simulink model "single_integrator_formation_control"  (R2021b)
settings: Solver=ode4  StartTime=0.0  StopTime=10  FixedStep=0.1  RelTol=1e-3
values from neighbouring files (symbols this model uses):
  A = A - diag(diag(A))    [formation_params.m]
  central_bot_idx = 5    [formation_params.m]
  init_positions = init_positions + init_position_perturbation    [formation_params.m]
  num_bots = 5    [formation_params.m]
  static_formation = [0.0, 0.0, 0.0 ... (first row only)    [formation_params.m]
libraries: robotcorelib x1
settings Model: Creator=root  LastModifiedBy=NEELAKSH SINGH

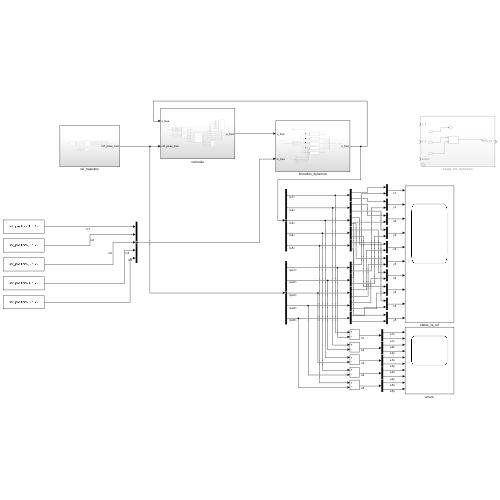
[thumbnail: Simulink's stored preview of the top-level diagram]
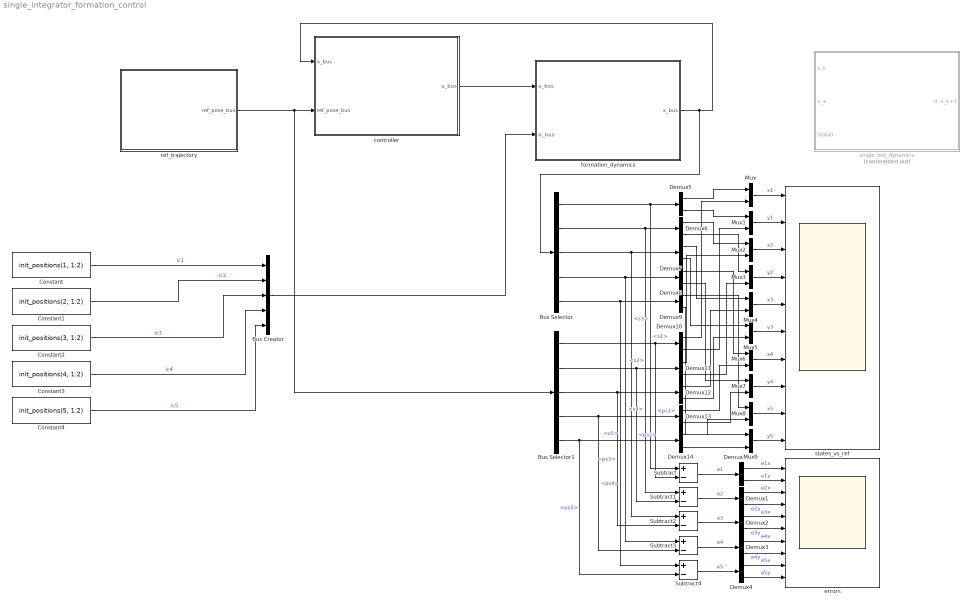
== system single_integrator_formation_control ==
  Bus Creator : BusCreator  Inputs=5
  Bus Selector : BusSelector  OutputSignals=s1,s2,s3,s4,s5
  Bus Selector1 : BusSelector  OutputSignals=ps1,ps2,ps3,ps4,ps5
  Constant : Constant  Value=init_positions(1, 1:2)
  Constant1 : Constant  Value=init_positions(2, 1:2)
  Constant2 : Constant  Value=init_positions(3, 1:2)
  Constant3 : Constant  Value=init_positions(4, 1:2)
  Constant4 : Constant  Value=init_positions(5, 1:2)
  Demux{,1..14} (15 alike) : Demux  Outputs=2
  Mux{,1..9} (10 alike) : Mux  Inputs=2
  Subtract{,1..4} (5 alike) : Sum  Inputs=+-
  controller : Subsystem
  errors : Scope  NumInputPorts=10
  formation_dynamics : Subsystem
  ref_trajectory : Subsystem
  single_bot_dynamics : Subsystem  Commented=on
  states_vs_ref : Scope  NumInputPorts=10
  wires:
  controller/1(u_bus) -> formation_dynamics/1(u_bus)
  formation_dynamics/1(x_bus) -> Bus Selector/1, controller/1(x_bus)
  Constant/1 -> Bus Creator/1  "ic1"
  Constant1/1 -> Bus Creator/2  "ic2"
  Constant2/1 -> Bus Creator/3  "ic3"
  Constant3/1 -> Bus Creator/4  "ic4"
  Constant4/1 -> Bus Creator/5  "ic5"
  Bus Creator/1 -> formation_dynamics/2(ic_bus)
  ref_trajectory/1(ref_pose_bus) -> Bus Selector1/1, controller/2(ref_pose_bus)
  Bus Selector/1 -> Demux5/1, Subtract/1  "<s1>"
  Bus Selector/2 -> Subtract1/1, Demux6/1  "<s2>"
  Bus Selector/3 -> Demux7/1, Subtract2/1  "<s3>"
  Bus Selector/4 -> Demux8/1, Subtract3/1  "<s4>"
  Bus Selector/5 -> Subtract4/1, Demux9/1  "<s5>"
  Bus Selector1/1 -> Demux10/1, Subtract/2  "<ps1>"
  Bus Selector1/2 -> Demux11/1, Subtract1/2  "<ps2>"
  Bus Selector1/3 -> Demux12/1, Subtract2/2  "<ps3>"
  Bus Selector1/4 -> Demux13/1, Subtract3/2  "<ps4>"
  Bus Selector1/5 -> Demux14/1, Subtract4/2  "<ps5>"
  Subtract4/1 -> Demux4/1  "e5"
  Subtract3/1 -> Demux3/1  "e4"
  Subtract2/1 -> Demux2/1  "e3"
  Subtract1/1 -> Demux1/1  "e2"
  Subtract/1 -> Demux/1  "e1"
  Demux/1 -> errors/1  "e1x"
  Demux4/2 -> errors/10  "e5y"
  Demux4/1 -> errors/9  "e5x"
  Demux3/1 -> errors/7  "e4x"
  Demux3/2 -> errors/8  "e4y"
  Demux2/2 -> errors/6  "e3y"
  Demux2/1 -> errors/5  "e3x"
  Demux1/2 -> errors/4  "e2y"
  Demux1/1 -> errors/3  "e2x"
  Demux/2 -> errors/2  "e1y"
  Demux5/1 -> Mux/1
  Demux10/1 -> Mux/2
  Demux5/2 -> Mux1/1
  Demux10/2 -> Mux1/2
  Demux6/1 -> Mux2/1
  Demux11/1 -> Mux2/2
  Demux6/2 -> Mux3/1
  Demux11/2 -> Mux3/2
  Demux7/1 -> Mux4/1
  Demux12/1 -> Mux4/2
  Demux7/2 -> Mux5/1
  Demux12/2 -> Mux5/2
  Demux8/1 -> Mux6/1
  Demux13/1 -> Mux6/2
  Demux8/2 -> Mux7/1
  Demux13/2 -> Mux7/2
  Demux9/1 -> Mux8/1
  Demux14/1 -> Mux8/2
  Demux9/2 -> Mux9/1
  Demux14/2 -> Mux9/2
  Mux/1 -> states_vs_ref/1  "x1"
  Mux1/1 -> states_vs_ref/2  "y1"
  Mux2/1 -> states_vs_ref/3  "x2"
  Mux3/1 -> states_vs_ref/4  "y2"
  Mux4/1 -> states_vs_ref/5  "x3"
  Mux5/1 -> states_vs_ref/6  "y3"
  Mux6/1 -> states_vs_ref/7  "x4"
  Mux7/1 -> states_vs_ref/8  "y4"
  Mux8/1 -> states_vs_ref/9  "x5"
  Mux9/1 -> states_vs_ref/10  "y5"

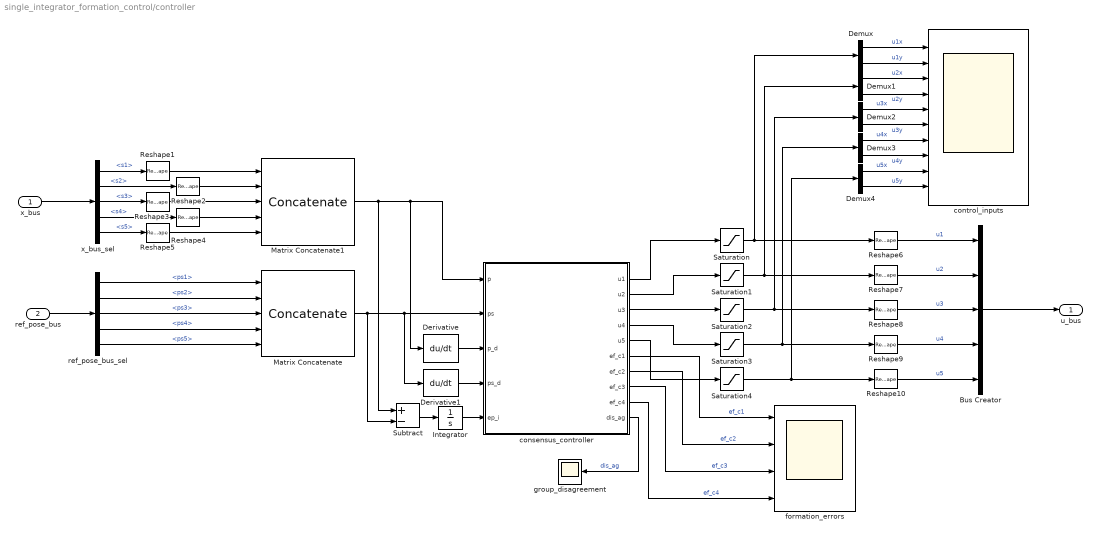
== system single_integrator_formation_control/controller ==
  x_bus : Inport
  ref_pose_bus : Inport  Port=2
  Bus Creator : BusCreator  Inputs=5
  Demux{,1..4} (5 alike) : Demux  Outputs=2
  Derivative : Derivative
  Derivative1 : Derivative
  Integrator : Integrator
  Matrix Concatenate : Concatenate  NumInputs=5  Mode=Multidimensional array  ConcatenateDimension=2
  Matrix Concatenate1 : Concatenate  NumInputs=5  Mode=Multidimensional array  ConcatenateDimension=2
  Reshape{1..10} (10 alike) : Reshape  OutputDimensionality=Column vector (2-D)
  Saturation{,1..4} (5 alike) : Saturate  UpperLimit=1  LowerLimit=-1
  Subtract : Sum  Inputs=+-
  consensus_controller : MATLAB Function  TreatAsAtomicUnit=on
  control_inputs : Scope  NumInputPorts=10
  formation_errors : Scope  NumInputPorts=4
  group_disagreement : Scope
  ref_pose_bus_sel : BusSelector  OutputSignals=ps1,ps2,ps3,ps4,ps5
  x_bus_sel : BusSelector  OutputSignals=s1,s2,s3,s4,s5
  u_bus : Outport
  wires:
  Bus Creator/1 -> u_bus/1
  consensus_controller/1(u1) -> Saturation/1
  consensus_controller/2(u2) -> Saturation1/1
  consensus_controller/3(u3) -> Saturation2/1
  consensus_controller/4(u4) -> Saturation3/1
  consensus_controller/5(u5) -> Saturation4/1
  x_bus_sel/1 -> Reshape1/1  "<s1>"
  x_bus_sel/2 -> Reshape2/1  "<s2>"
  x_bus_sel/3 -> Reshape3/1  "<s3>"
  x_bus_sel/4 -> Reshape4/1  "<s4>"
  x_bus_sel/5 -> Reshape5/1  "<s5>"
  ref_pose_bus/1 -> ref_pose_bus_sel/1
  Reshape6/1 -> Bus Creator/1  "u1"
  Reshape7/1 -> Bus Creator/2  "u2"
  Reshape8/1 -> Bus Creator/3  "u3"
  Reshape9/1 -> Bus Creator/4  "u4"
  Reshape10/1 -> Bus Creator/5  "u5"
  consensus_controller/9(ef_c4) -> formation_errors/4  "ef_c4"
  consensus_controller/6(ef_c1) -> formation_errors/1  "ef_c1"
  consensus_controller/7(ef_c2) -> formation_errors/2  "ef_c2"
  consensus_controller/8(ef_c3) -> formation_errors/3  "ef_c3"
  Demux4/2 -> control_inputs/10  "u5y"
  Demux/1 -> control_inputs/1  "u1x"
  Demux/2 -> control_inputs/2  "u1y"
  Demux1/1 -> control_inputs/3  "u2x"
  Demux1/2 -> control_inputs/4  "u2y"
  Demux2/1 -> control_inputs/5  "u3x"
  Demux2/2 -> control_inputs/6  "u3y"
  Demux3/1 -> control_inputs/7  "u4x"
  Demux3/2 -> control_inputs/8  "u4y"
  Demux4/1 -> control_inputs/9  "u5x"
  Saturation/1 -> Demux/1, Reshape6/1
  Saturation1/1 -> Demux1/1, Reshape7/1
  Saturation2/1 -> Demux2/1, Reshape8/1
  Saturation3/1 -> Demux3/1, Reshape9/1
  Saturation4/1 -> Demux4/1, Reshape10/1
  ref_pose_bus_sel/1 -> Matrix Concatenate/1  "<ps1>"
  ref_pose_bus_sel/2 -> Matrix Concatenate/2  "<ps2>"
  ref_pose_bus_sel/3 -> Matrix Concatenate/3  "<ps3>"
  ref_pose_bus_sel/4 -> Matrix Concatenate/4  "<ps4>"
  ref_pose_bus_sel/5 -> Matrix Concatenate/5  "<ps5>"
  Matrix Concatenate/1 -> Subtract/2, Derivative1/1, consensus_controller/2(ps)
  Reshape2/1 -> Matrix Concatenate1/2
  Reshape4/1 -> Matrix Concatenate1/4
  Reshape1/1 -> Matrix Concatenate1/1
  Reshape3/1 -> Matrix Concatenate1/3
  Reshape5/1 -> Matrix Concatenate1/5
  Matrix Concatenate1/1 -> consensus_controller/1(p), Derivative/1, Subtract/1
  x_bus/1 -> x_bus_sel/1
  Derivative/1 -> consensus_controller/3(p_d)
  Derivative1/1 -> consensus_controller/4(ps_d)
  Subtract/1 -> Integrator/1
  Integrator/1 -> consensus_controller/5(ep_i)
  consensus_controller/10(dis_ag) -> group_disagreement/1  "dis_ag"

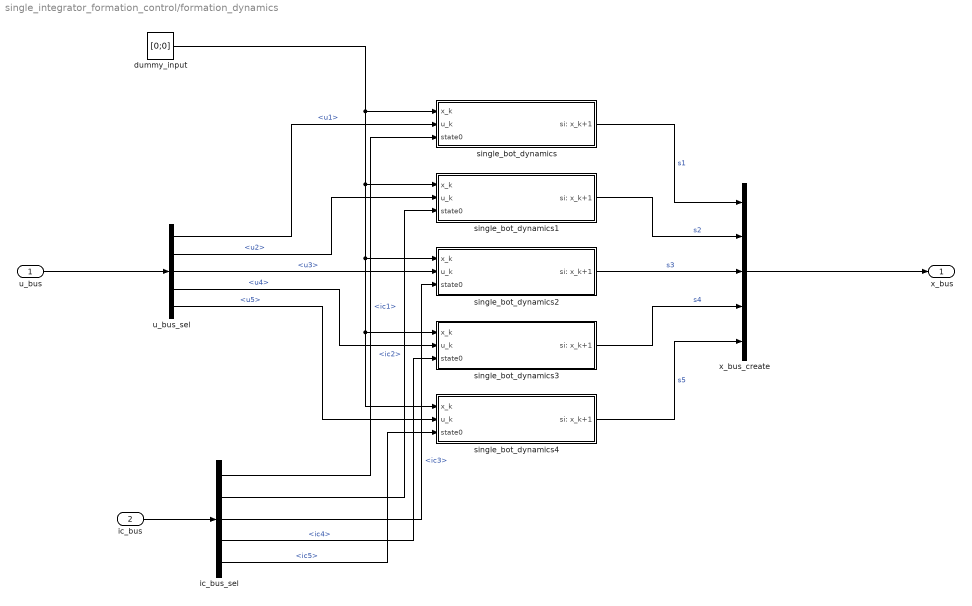
== system single_integrator_formation_control/formation_dynamics ==
  u_bus : Inport
  ic_bus : Inport  Port=2
  dummy_input : Constant  Value=[0;0]
  ic_bus_sel : BusSelector  OutputSignals=ic1,ic2,ic3,ic4,ic5
  single_bot_dynamics : Subsystem
  single_bot_dynamics1 : Subsystem
  single_bot_dynamics2 : Subsystem
  single_bot_dynamics3 : Subsystem
  single_bot_dynamics4 : Subsystem
  u_bus_sel : BusSelector  OutputSignals=u1,u2,u3,u4,u5
  x_bus_create : BusCreator  Inputs=5
  x_bus : Outport
  wires:
  u_bus_sel/1 -> single_bot_dynamics/2(u_k)  "<u1>"
  u_bus_sel/2 -> single_bot_dynamics1/2(u_k)  "<u2>"
  u_bus_sel/3 -> single_bot_dynamics2/2(u_k)  "<u3>"
  u_bus_sel/4 -> single_bot_dynamics3/2(u_k)  "<u4>"
  u_bus_sel/5 -> single_bot_dynamics4/2(u_k)  "<u5>"
  single_bot_dynamics1/1(si: x_k+1) -> x_bus_create/2  "s2"
  single_bot_dynamics2/1(si: x_k+1) -> x_bus_create/3  "s3"
  single_bot_dynamics3/1(si: x_k+1) -> x_bus_create/4  "s4"
  single_bot_dynamics4/1(si: x_k+1) -> x_bus_create/5  "s5"
  ic_bus/1 -> ic_bus_sel/1
  ic_bus_sel/1 -> single_bot_dynamics/3(state0)  "<ic1>"
  ic_bus_sel/2 -> single_bot_dynamics1/3(state0)  "<ic2>"
  ic_bus_sel/3 -> single_bot_dynamics2/3(state0)  "<ic3>"
  ic_bus_sel/4 -> single_bot_dynamics3/3(state0)  "<ic4>"
  ic_bus_sel/5 -> single_bot_dynamics4/3(state0)  "<ic5>"
  u_bus/1 -> u_bus_sel/1
  x_bus_create/1 -> x_bus/1
  single_bot_dynamics/1(si: x_k+1) -> x_bus_create/1  "s1"
  dummy_input/1 -> single_bot_dynamics4/1(x_k), single_bot_dynamics3/1(x_k), single_bot_dynamics2/1(x_k), single_bot_dynamics1/1(x_k), single_bot_dynamics/1(x_k)

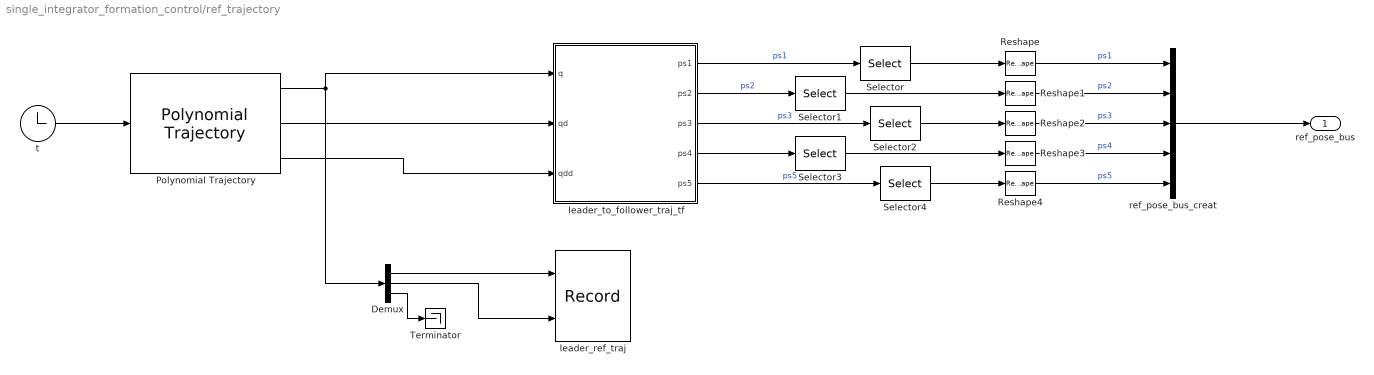
== system single_integrator_formation_control/ref_trajectory ==
  Demux : Demux  Outputs=3
  Polynomial Trajectory : robotcorelib/Polynomial Trajectory  WaypointSource=Internal  Waypoints=waypoints  TimePoints=time_points  TimeInterval=[ 1, 4 ]  Method=Cubic Polynomial  ParameterSource=Internal  VelocityBoundaryCondition=velocity_conditions  AccelerationBoundaryCondition=zeros( 2, 5 )  SimulateUsing=Interpreted execution
  Reshape{,1..4} (5 alike) : Reshape  OutputDimensionality=Column vector (2-D)
  Selector{,1..4} (5 alike) : Selector  InputPortWidth=3  IndexOptions=Index vector (dialog)  Indices=[1 2]  OutputSizes=1
  Terminator : Terminator
  leader_ref_traj : Record  FileSettingsInternal="{\"entries\":[{\"content\":{\"excelSettings\":{\"content\":{},\"type\":\"Streamout.ExcelSettings\"}},\"type\":\"Streamout.FileSettingStorage\",\"uuid\":\"e7b4e02a-8a6c-4c28-bff8-32dd845a5106\"}],\"packageUris\":[\"http://schema.mathworks.com/mf0/streamout_blocks/R2020a\"],\"version\":\"1.0\"}"  Layout=[1 1]  SignalsInternal="{\"entries\":[{\"content\":{\"signals\":[{\"content\":{\"blockPath\":[\"single_integrator_formation_control/ref_trajectory/leader_ref_traj\"],\"channel\":[],\"dimensions\":[1,1],\"domain\":\"single_integrator_formation_control/ref_trajectory/leader_ref_traj\",\"lineColor\":\"#a2142f\",\"plots\":[1],\"port\":1,\"sid\":[\"\"],\"signalID\":8769,\"signalName\":\"Demux:1\"},\"type\":\"RecordBlkView.Signal\",\"uuid\":\"6b5f94f3-8821-4aca-bcdf-331b5f50b77f\"},{\"content\":{\"blockPath\":[\"single_integrator_formation_control/ref_trajectory/leader_ref_traj\"],\"channel\":[],\"dimensions\":[1,1],\"domain\":\"single_integrator_formation_control/ref_trajectory/leader_ref_traj\",\"lineColor\":\"#139fff\",\"plots\":[1],\"port\":2,\"sid\":[\"\"],\"signalID\":8773,\"signalName\":\"Demux:2\"},\"type\":\"RecordBlkView.Signal\",\"uuid\":\"b17d3734-1416-4d17-a2be-2707baf58851\"}]},\"type\":\"RecordBlkView.InputSignals\",\"uuid\":\"13d1e91a-ab3f-42d2-9c1f-47b71bbe905e\"}],\"packageUris\":[\"http://schema.mathworks.com/mf0/streamout_blocks/R2020a\"],\"version\":\"1.0\"}"  VisualizationBindings="{\"xyplotplugin\":{\"info\":[{\"series\":[{\"bindingParametersList\":[{\"parameter\":\"X-Axis\",\"signalID\":8769,\"signalName\":\"Demux:1\"},{\"parameter\":\"Y-Axis\",\"signalID\":8773,\"signalName\":\"Demux:2\"}],\"seriesID\":26954}],\"subplotID\":1}]}}"  CompatibilityTag=XY  st=-1
  leader_to_follower_traj_tf : MATLAB Function  TreatAsAtomicUnit=on
  ref_pose_bus_creat : BusCreator  Inputs=5
  t : Clock
  ref_pose_bus : Outport
  wires:
  ref_pose_bus_creat/1 -> ref_pose_bus/1
  t/1 -> Polynomial Trajectory/1
  Polynomial Trajectory/1 -> Demux/1, leader_to_follower_traj_tf/1(q)
  Polynomial Trajectory/2 -> leader_to_follower_traj_tf/2(qd)
  Polynomial Trajectory/3 -> leader_to_follower_traj_tf/3(qdd)
  Demux/1 -> leader_ref_traj/1
  Demux/2 -> leader_ref_traj/2
  leader_to_follower_traj_tf/1(ps1) -> Selector/1  "ps1"
  leader_to_follower_traj_tf/3(ps3) -> Selector2/1  "ps3"
  leader_to_follower_traj_tf/5(ps5) -> Selector4/1  "ps5"
  Reshape/1 -> ref_pose_bus_creat/1  "ps1"
  Reshape1/1 -> ref_pose_bus_creat/2  "ps2"
  Reshape2/1 -> ref_pose_bus_creat/3  "ps3"
  Reshape3/1 -> ref_pose_bus_creat/4  "ps4"
  Reshape4/1 -> ref_pose_bus_creat/5  "ps5"
  Selector/1 -> Reshape/1
  leader_to_follower_traj_tf/2(ps2) -> Selector1/1  "ps2"
  Selector1/1 -> Reshape1/1
  Selector2/1 -> Reshape2/1
  Selector3/1 -> Reshape3/1
  Selector4/1 -> Reshape4/1
  Demux/3 -> Terminator/1
  leader_to_follower_traj_tf/4(ps4) -> Selector3/1

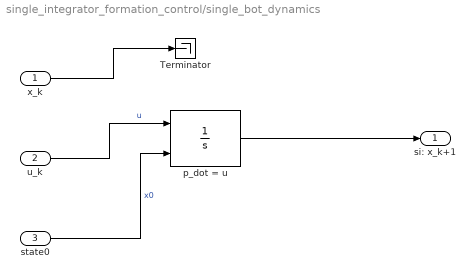
== system single_integrator_formation_control/single_bot_dynamics ==
  x_k : Inport
  u_k : Inport  Port=2
  state0 : Inport  Port=3
  Terminator : Terminator
  p_dot = u : Integrator  InitialConditionSource=external
  si: x_k+1 : Outport
  wires:
  x_k/1 -> Terminator/1
  u_k/1 -> p_dot = u/1  "u"
  state0/1 -> p_dot = u/2  "x0"
  p_dot = u/1 -> si: x_k+1/1

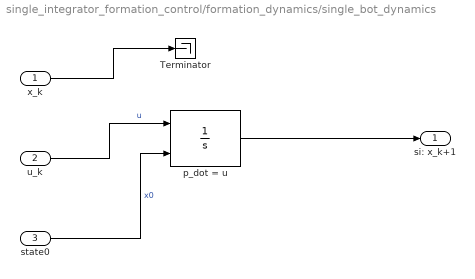
== system single_integrator_formation_control/formation_dynamics/single_bot_dynamics ==
  x_k : Inport
  u_k : Inport  Port=2
  state0 : Inport  Port=3
  Terminator : Terminator
  p_dot = u : Integrator  InitialConditionSource=external
  si: x_k+1 : Outport
  wires:
  x_k/1 -> Terminator/1
  u_k/1 -> p_dot = u/1  "u"
  state0/1 -> p_dot = u/2  "x0"
  p_dot = u/1 -> si: x_k+1/1

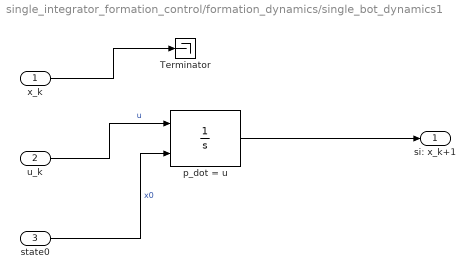
== system single_integrator_formation_control/formation_dynamics/single_bot_dynamics1 ==
  x_k : Inport
  u_k : Inport  Port=2
  state0 : Inport  Port=3
  Terminator : Terminator
  p_dot = u : Integrator  InitialConditionSource=external
  si: x_k+1 : Outport
  wires:
  x_k/1 -> Terminator/1
  u_k/1 -> p_dot = u/1  "u"
  state0/1 -> p_dot = u/2  "x0"
  p_dot = u/1 -> si: x_k+1/1

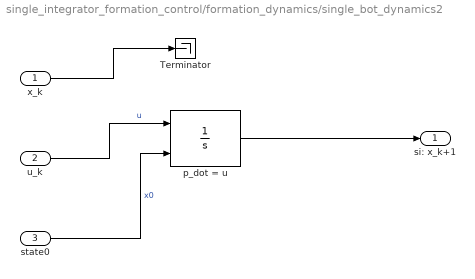
== system single_integrator_formation_control/formation_dynamics/single_bot_dynamics2 ==
  x_k : Inport
  u_k : Inport  Port=2
  state0 : Inport  Port=3
  Terminator : Terminator
  p_dot = u : Integrator  InitialConditionSource=external
  si: x_k+1 : Outport
  wires:
  x_k/1 -> Terminator/1
  u_k/1 -> p_dot = u/1  "u"
  state0/1 -> p_dot = u/2  "x0"
  p_dot = u/1 -> si: x_k+1/1

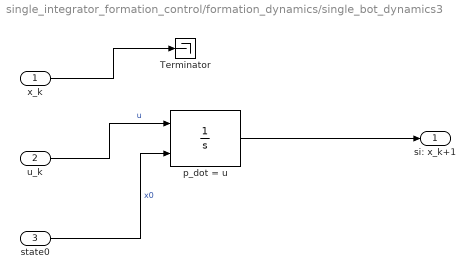
== system single_integrator_formation_control/formation_dynamics/single_bot_dynamics3 ==
  x_k : Inport
  u_k : Inport  Port=2
  state0 : Inport  Port=3
  Terminator : Terminator
  p_dot = u : Integrator  InitialConditionSource=external
  si: x_k+1 : Outport
  wires:
  x_k/1 -> Terminator/1
  u_k/1 -> p_dot = u/1  "u"
  state0/1 -> p_dot = u/2  "x0"
  p_dot = u/1 -> si: x_k+1/1

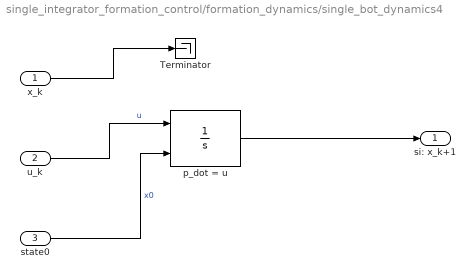
== system single_integrator_formation_control/formation_dynamics/single_bot_dynamics4 ==
  x_k : Inport
  u_k : Inport  Port=2
  state0 : Inport  Port=3
  Terminator : Terminator
  p_dot = u : Integrator  InitialConditionSource=external
  si: x_k+1 : Outport
  wires:
  x_k/1 -> Terminator/1
  u_k/1 -> p_dot = u/1  "u"
  state0/1 -> p_dot = u/2  "x0"
  p_dot = u/1 -> si: x_k+1/1

== matlab function single_integrator_formation_control/ref_trajectory/leader_to_follower_traj_tf ==
  data: q input; ps1 output; ps2 output; ps3 output; ps4 output; ps5 output; qd input; qdd input; tf_list parameter
function [ps1, ps2, ps3, ps4, ps5] = l2f_traj_tf(q, qd, qdd, tf_list)
ps1 = zeros(size(q));
ps2 = zeros(size(q));
ps3 = zeros(size(q));
ps4 = zeros(size(q));
ps5 = zeros(size(q));
ps1_t = tf_list(:,:,1)*cart2hom(q')';
ps2_t = tf_list(:,:,2)*cart2hom(q')';
ps3_t = tf_list(:,:,3)*cart2hom(q')';
ps4_t = tf_list(:,:,4)*cart2hom(q')';
ps1 = ps1_t(1:3);
ps2 = ps2_t(1:3);
ps3 = ps3_t(1:3);
ps4 = ps4_t(1:3);
ps5 = q;

== matlab function single_integrator_formation_control/controller/consensus_controller ==
  data: p input; u1 output; u2 output; u3 output; u4 output; ps input; p_d input; ps_d input; ep_i input; u5 output; A parameter; num_bots parameter; ef_c1 output; ef_c2 output; ef_c3 output; ef_c4 output; central_bot_idx parameter; static_formation parameter; dis_ag output
function [u1,u2,u3,u4,u5, ef_c1, ef_c2, ef_c3, ef_c4, dis_ag] = consensus_controller(p, ps, p_d, ps_d, ep_i, A, num_bots, central_bot_idx, static_formation)
%% FLAGS
USE_PID_CONTROLLER = false;
USE_CONSENSUS_WEIGHT = false; % INSTEAD OF USING THIS, IT IS PREFERRED TO CHANGE ADJACENCY MATRIX INSTEAD.
%% Setting Parameters
u_dim = [2,1];
u = zeros(u_dim(1), u_dim(2), num_bots);
p_dim = size(p(:,1));
% ps = horzcat(ps1,ps2,ps3,ps4,ps5);
% p = horzcat(s1,s2,s3,s4,s5);

beta = 1;
W_P_DOT = 1;
kp = 2;
kd = 0.1;
ki = 0.5;
consensus_weight = 1.5;

%% Using the behavior consensus law

if ~USE_CONSENSUS_WEIGHT
    consensus_weight = 1;
end
%%% ERRATA: Forgot to add the p_dot term last time to the LHS of the final
%%% control law in the consensus algorithm. 
if ~USE_PID_CONTROLLER
    for i=1:1:num_bots
        consensus_term = zeros(p_dim(1), p_dim(2));
        for j = 1:1:num_bots
            consensus_term = consensus_term + A(i,j)*((p(:,i) - p(:,j)) - (ps(:,i) - ps(:,j)));
        end
        backstep_term = beta*(p(:,i) - ps(:,i));
        u(:,:,i) = W_P_DOT*p_d(:,i) - backstep_term - consensus_weight*consensus_term;
    end
end

if USE_PID_CONTROLLER
    for i=1:1:num_bots
        consensus_term = zeros(p_dim(1), p_dim(2));
        for j = 1:1:num_bots
            consensus_term = consensus_term + A(i,j)*((p(:,i) - ps(:,i)) - (p(:,j) - ps(:,j)));
        end
        PID_term = kp*(p(:,i) - ps(:,i)) + kd*(p_d(:,i) - ps_d(:,i)) + ki*ep_i(:,i);
        u(:,:,i) = -PID_term - consensus_weight*consensus_term;
    end
end
%% Unpacking the u vector of control_inputs.
u1 = u(:,:,1);
u2 = u(:,:,2);
u3 = u(:,:,3);
u4 = u(:,:,4);
u5 = u(:,:,5);

%% Calculating the formation errors
ef_idx_vec = zeros(num_bots, 2);
ef_idx_vec(:,1) = central_bot_idx;
ef_vec = zeros(p_dim(1), p_dim(2), num_bots);
dis_ag = 0;

for i=1:num_bots
    ef_vec(:,:,i) = (p(:, i) - p(:, central_bot_idx)) - (static_formation(i,1:2) - static_formation(central_bot_idx,1:2))';
    for j=1:num_bots
        dis_ag = dis_ag + 0.5*A(i,j)*(norm((p(:,i) - ps(:,i)) - (p(:,j) - ps(:,j)))^2);
    end
end

ef_c1 = ef_vec(:,:,1);
ef_c2 = ef_vec(:,:,2);
ef_c3 = ef_vec(:,:,3);
ef_c4 = ef_vec(:,:,4);
